simulink model "openloopstatetraj1"  (Simulink 8.6)
settings: Solver=ode1  StartTime=0.0  StopTime=stoptime  FixedStep=dt  RelTol=1e-3
values from neighbouring files (symbols this model uses):
  Ahat = A    [olsleaderfollowertest2.m]    (also in olsleaderfollowertest3.m; simpleexamplesimulationresults.mat = [-1  1; 0  -1]; test.mat = [-1  1; 0  -1])
  Bhat = [B1 B2 F]    [olsleaderfollowertest2.m]    (also in olsleaderfollowertest3.m; simpleexamplesimulationresults.mat = [0  0  1; 1  1  1]; test.mat = [0  0  1; 1  1  1])
  Chat = eye(n,n)    [olsleaderfollowertest2.m]    (also in olsleaderfollowertest3.m; simpleexamplesimulationresults.mat = [1  0; 0  1]; test.mat = [1  0; 0  1])
  Dhat = zeros(n,length(Bhat))    [olsleaderfollowertest2.m]    (also in olsleaderfollowertest3.m; simpleexamplesimulationresults.mat = [0  0  0; 0  0  0]; test.mat = [0  0  0; 0  0  0])
  dt = 1e-2    (= 0.01)    [olsleaderfollowertest2.m]    (also in olsleaderfollowertest3.m; simpleexamplesimulationresults.mat; test.mat)
  x0 = [4 3]    [simpleexamplesimulationresults.mat]    (also in simplemodel4.m = [4 3].'; test.mat)
undefined symbols (not defined in the file): randseed, W
settings Model: Creator=Firdous  LastModifiedBy=Firdous
settings DataIOCC: LimitDataPoints=off  SaveState=on  ReturnWorkspaceOutputs=on
settings DebuggingCC: FcnCallInpInsideContextMsg=EnableAllAsWarning

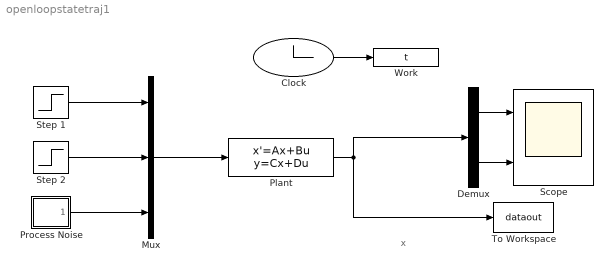
== system openloopstatetraj1 ==
  note: x
  Clock : Clock
  Demux : Demux  Outputs=2
  Mux : Mux  Inputs=3
  Plant : StateSpace  A=Ahat  B=Bhat  C=Chat  D=Dhat  X0=x0
  Process Noise : Subsystem  mask(Continuous White Noise.){Cov=W, Ts=dt, seed=randseed}
      mask prompts: Cov "Noise Variance:"; Ts "Sample Time:"
      mask help:
      | White noise for continuous (s-domain) systems.
      | Band-limited using zero-order-hold.
      mask Help: Implemented using white noise into Zero Order Hold block. For faster simulation set sample time to highest value possible but in accordance with the fastest dynamics of system.
      mask Display: plot(1:20,rand(size(1:20)))
  Scope : Scope  NumInputPorts=2
  Step 1 : Step  Time=0  SampleTime=dt
  Step 2 : Step  Time=0  SampleTime=dt
  To Workspace : ToWorkspace  VariableName=dataout  SampleTime=-1
  Work : ToWorkspace  VariableName=t
      settings: MaxDataPoints=stoptime
  wires:
  Clock/1 -> Work/1
  Plant/1 -> To Workspace/1, Demux/1
  Mux/1 -> Plant/1
  Demux/1 -> Scope/1
  Step 2/1 -> Mux/2
  Process Noise/1(out_1) -> Mux/3
  Step 1/1 -> Mux/1
  Demux/2 -> Scope/2

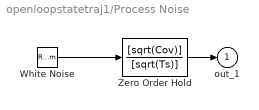
== system openloopstatetraj1/Process Noise ==
  White Noise : RandomNumber  Seed=seed  SampleTime=dt
  Zero Order Hold : DiscreteTransferFcn  Numerator=[sqrt(Cov)]  Denominator=[sqrt(Ts)]  SampleTime=Ts
  out_1 : Outport
  wires:
  Zero Order Hold/1 -> out_1/1
  White Noise/1 -> Zero Order Hold/1
